simulink model "MDL3_Longitudinal_Vehicle_Model_Lib_Mask"  (R2025b)
settings: Solver=VariableStepAuto  StartTime=0.0  StopTime=20  MaxStep=1/100  MinStep=1/1000  RelTol=1e-3
InitFcn:
  | mdl2_longitudinal_vehicle_init_params
undefined symbols (not defined in the file): F_T, m
libraries: Longintudinal_Vehicle_Opposing_Force_Components_Lib x3
settings Model: Creator=rkash  LastModifiedBy=rkash

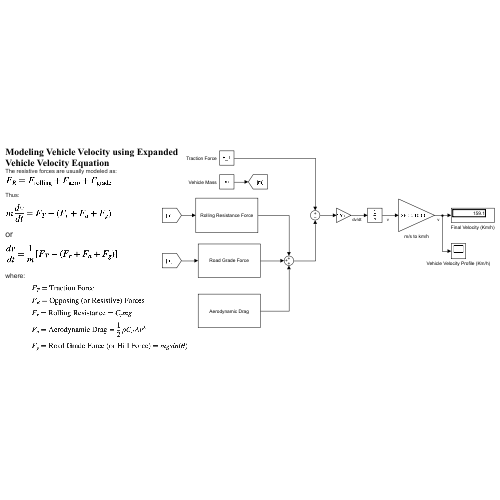
[thumbnail: Simulink's stored preview of the top-level diagram]
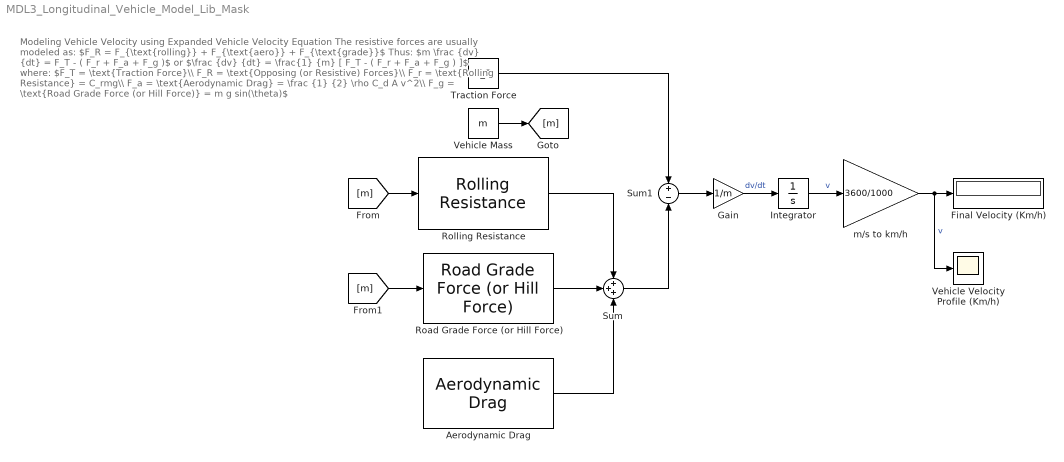
== system MDL3_Longitudinal_Vehicle_Model_Lib_Mask ==
  note: Modeling Vehicle Velocity using Expanded Vehicle Velocity Equation
      | The resistive forces are usually modeled as:
      | $F_R = F_{\text{rolling}} + F_{\text{aero}} + F_{\text{grade}}$
      | Thus:
      | $m \frac {dv} {dt} = F_T - ( F_r + F_a + F_g )$
      | or
      | $\frac {dv} {dt} = \frac{1} {m} [ F_T - ( F_r + F_a + F_g ) ]$
      | where:
      | $F_T = \text{Traction Force}\\ F_R = \text{Opposing (or Resistive) Forces}\\ F_r = \text{Rolling Resistance} = C_rmg\\ F_a = \text{Aerodynamic Drag} = \frac {1} {2} \rho C_d A v^2\\ F_g = \text{Road Grade Force (or Hill Force)} = m g sin(\theta)$
  Aerodynamic Drag : Longintudinal_Vehicle_Opposing_Force_Components_Lib/Aerodynamic Drag  rho=1.225  C_d=0.32  A=2.2  v=20
  Final Velocity (Km/h) : Display
  Gain : Gain  Gain=1/m
  Integrator : Integrator
  Road Grade Force (or Hill Force) : Longintudinal_Vehicle_Opposing_Force_Components_Lib/Road Grade Force (or Hill Force)  g=9.81  theta=0
  Rolling Resistance : Longintudinal_Vehicle_Opposing_Force_Components_Lib/Rolling Resistance  g=9.81  C_r=0.015
  Sum : Sum  Inputs=+++
  Sum1 : Sum  Inputs=+-
  Traction Force : Constant  Value=F_T
  Vehicle Mass : Constant  Value=m
  Vehicle Velocity Profile (Km/h) : Scope
      settings: ActiveDisplayYMinimum=-1  ActiveDisplayYMaximum=1
  m/s to km/h : Gain  Gain=3600/1000
  wires:
  Rolling Resistance/1 -> Sum/1
  Road Grade Force (or Hill Force)/1 -> Sum/2
  Aerodynamic Drag/1 -> Sum/3
  Traction Force/1 -> Sum1/1
  Sum/1 -> Sum1/2
  Sum1/1 -> Gain/1
  Gain/1 -> Integrator/1  "dv/dt"
  Integrator/1 -> m/s to km/h/1  "v"
  m/s to km/h/1 -> Vehicle Velocity Profile (Km/h)/1, Final Velocity (Km/h)/1  "v"
  Vehicle Mass/1 -> [m]
  [m] -> Rolling Resistance/1
  [m] -> Road Grade Force (or Hill Force)/1
